simulink model "problema2"  (R2023b)
settings: Solver=VariableStepAuto  StartTime=0.0  StopTime=10.0  RelTol=1e-3
values from neighbouring files (symbols this model uses):
  T = 1/1000    (= 0.001)    [problema1.m]    (also in problema2.m = 0.1; problema5.m = [0.5*10^-3])
settings Model: Creator=Lenovo  LastModifiedBy=Lenovo

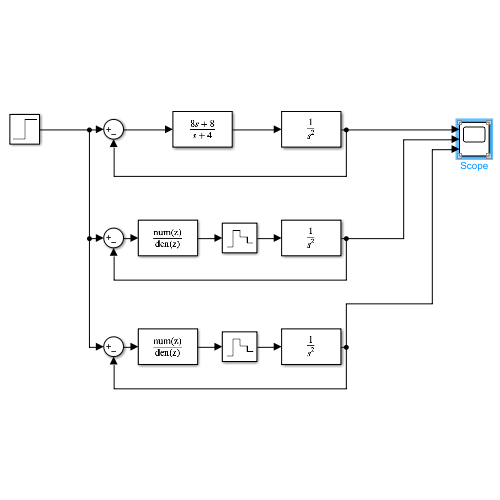
[thumbnail: Simulink's stored preview of the top-level diagram]
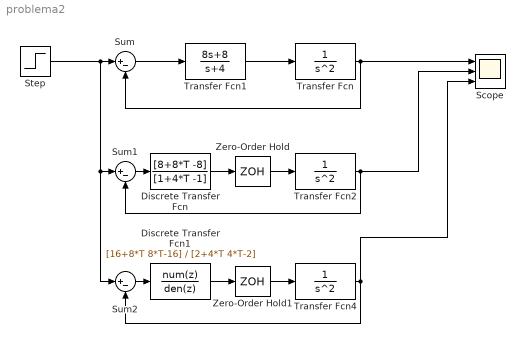
== system problema2 ==
  Discrete Transfer Fcn : DiscreteTransferFcn  Numerator=[8+8*T -8]  Denominator=[1+4*T -1]
  Discrete Transfer Fcn1 : DiscreteTransferFcn  Numerator=[16+8*T 8*T-16]  Denominator=[2+4*T 4*T-2]
  Scope : Scope  NumInputPorts=3
  Step : Step  SampleTime=0
  Sum : Sum  Inputs=|+-
  Sum1 : Sum  Inputs=|+-
  Sum2 : Sum  Inputs=|+-
  Transfer Fcn : TransferFcn  Denominator=[1 0 0]
  Transfer Fcn1 : TransferFcn  Numerator=[8 8]  Denominator=[1 4]
  Transfer Fcn2 : TransferFcn  Denominator=[1 0 0]
  Transfer Fcn4 : TransferFcn  Denominator=[1 0 0]
  Zero-Order Hold : ZeroOrderHold  SampleTime=T
  Zero-Order Hold1 : ZeroOrderHold  SampleTime=T
  wires:
  Transfer Fcn1/1 -> Transfer Fcn/1
  Sum/1 -> Transfer Fcn1/1
  Transfer Fcn/1 -> Sum/2, Scope/1
  Step/1 -> Sum1/1, Sum2/1, Sum/1
  Transfer Fcn2/1 -> Sum1/2, Scope/2
  Transfer Fcn4/1 -> Sum2/2, Scope/3
  Sum1/1 -> Discrete Transfer Fcn/1
  Discrete Transfer Fcn/1 -> Zero-Order Hold/1
  Zero-Order Hold/1 -> Transfer Fcn2/1
  Sum2/1 -> Discrete Transfer Fcn1/1
  Discrete Transfer Fcn1/1 -> Zero-Order Hold1/1
  Zero-Order Hold1/1 -> Transfer Fcn4/1
